simulink model "family_5_variant_2_AR_Drone_Host_Receive"  (R2014a)
settings: Solver=FixedStepDiscrete  StartTime=0.0  StopTime=inf  FixedStep=1/400  RelTol=1e-3
libraries: vrlib x3, dspnetwork x3, aerolibtransform2 x3, aerolibutil x1
settings Model: Creator=nraman  LastModifiedBy=Raphaël

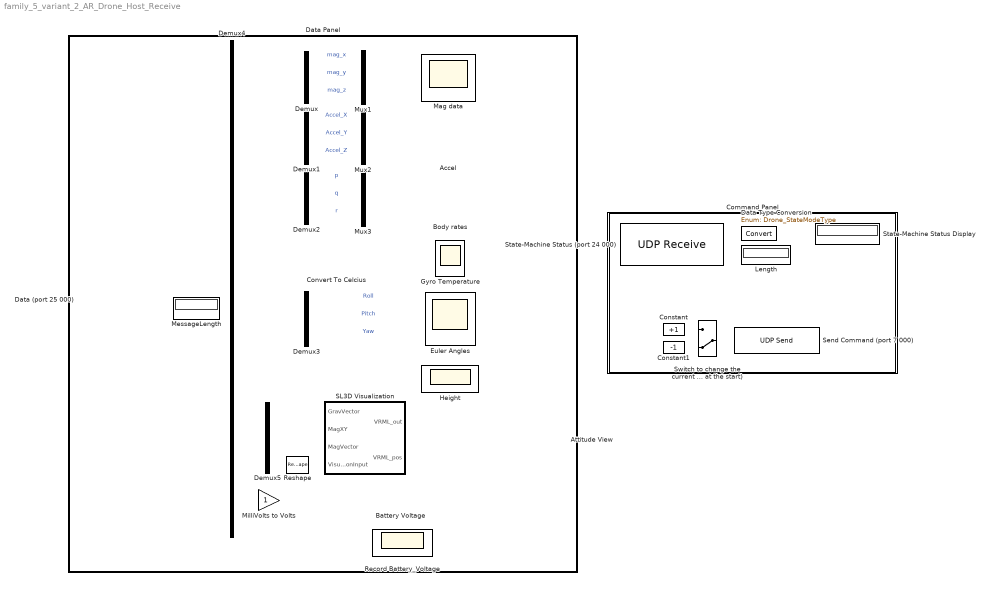
== system family_5_variant_2_AR_Drone_Host_Receive ==
  Accel : Scope
      settings: ShowLegends=on  TimeRange=100  YMin=2025  YMax=2575  SaveName=Accel
  Attitude View : vrlib/VR Sink  InstantiateOnLoad=on  SampleTime=-1  ViewEnable=on  RemoteChange=off  RemoteView=off  FieldsWritten=Drone.rotation.4.1.1.double#Drone.translation.3.1.1.double  WorldFileName=myDrone3.wrl  AutoView=off  VideoDimensions=[]  AllowVariableSize=off
  Battery Voltage : Display
  Body rates : Scope
      settings: ShowLegends=on  TimeRange=90  YMin=-45  YMax=35  SaveName=Gyro
  Command Panel : Subsystem
  Constant : Constant  Value=+1
  Constant1 : Constant  Value=-1
  Convert To Celcius : Subsystem
  Data (port 25 000) : dspnetwork/UDP Receive  localURL='0.0.0.0'  localPort=25000  remoteURL='192.168.1.1'  remotePort=-1  recvBufferSize=8192  dims=34  signalDatatype=double  isVarSize=off  showBlockingTime=off  blockingTime=0  sampletime=2/400
  Data Panel : Subsystem
  Data Type Conversion : DataTypeConversion  OutDataTypeStr=Enum: Drone_StateModeType
  Demux{,1..3} (4 alike) : Demux  Outputs=3
  Demux4 : Demux  Outputs=[3 3 3 1 3 2 18 1]
  Demux5 : Demux  Outputs=[3 3 3 9]
  Euler Angles : Scope  NumInputPorts=3
      settings: TimeRange=160  YMin=-1.04~-0.28~4.15  YMax=-0.87~-0.18~4.95  SaveName=EulerAngles
  Gyro Temperature : Scope
      settings: ShowLegends=on  TimeRange=100  YMin=47.5  YMax=82.5  SaveName=TempMeasure
  Height : Scope
      settings: YMin=-30  YMax=150  SaveName=RecordedHeight
  Length : Display
  Mag data : Scope
      settings: ShowLegends=on  TimeRange=100  YMin=-240  YMax=-30  SaveName=MagData
  MessageLength : Display
  MilliVolts to Volts : Gain
  Mux1 : Mux  Inputs=3
  Mux2 : Mux  Inputs=3
  Mux3 : Mux  Inputs=3
  Record Battery_Voltage : Scope
      settings: YMin=12.395  YMax=12.455
  Reshape : Reshape  OutputDimensionality=Customize  OutputDimensions=[3,3]
  SL3D Visualization : Subsystem
  Send Command (port 7 000) : dspnetwork/UDP Send  remoteURL='192.168.1.1'  remotePort=6000  localURL='0.0.0.0'  localPortSource=Automatically determine  localPort=-1  sampletime=-1  blockPlatform=LINUX  separateLengthPort=0
  State-Machine Status (port 24 000) : dspnetwork/UDP Receive  localURL='0.0.0.0'  localPort=24000  remoteURL='192.168.1.1'  remotePort=-1  recvBufferSize=100  dims=1  signalDatatype=int8  isVarSize=off  showBlockingTime=on  blockingTime=0.05  sampletime=1/400  blockPlatform=LINUX
  State-Machine Status Display : Display
  Switch to change the current Drone State (it has to be down at the start) : ManualSwitch  CurrentSetting=0
  wires:
  Demux4/1 -> Demux/1
  Demux/1 -> Mux1/1  "mag_x"
  Demux/2 -> Mux1/2  "mag_y"
  Demux/3 -> Mux1/3  "mag_z"
  Mux1/1 -> Mag data/1
  Demux2/1 -> Mux3/1  "p"
  Demux2/2 -> Mux3/2  "q"
  Mux3/1 -> Body rates/1
  Demux2/3 -> Mux3/3  "r"
  Demux4/3 -> Demux2/1
  Demux1/1 -> Mux2/1  "Accel_X"
  Demux1/2 -> Mux2/2  "Accel_Y"
  Mux2/1 -> Accel/1
  Demux1/3 -> Mux2/3  "Accel_Z"
  Demux4/2 -> Demux1/1
  Demux3/1 -> Euler Angles/1  "Roll"
  Demux3/2 -> Euler Angles/2  "Pitch"
  Demux4/5 -> Demux3/1
  Data (port 25 000)/1 -> Demux4/1
  MilliVolts to Volts/1 -> Battery Voltage/1, Record Battery_Voltage/1
  Demux3/3 -> Euler Angles/3  "Yaw"
  Data (port 25 000)/2 -> MessageLength/1
  State-Machine Status (port 24 000)/1 -> Data Type Conversion/1
  Data Type Conversion/1 -> State-Machine Status Display/1
  State-Machine Status (port 24 000)/2 -> Length/1
  Demux4/8 -> MilliVolts to Volts/1
  Demux4/4 -> Convert To Celcius/1(In1)
  Convert To Celcius/1(Out1) -> Gyro Temperature/1
  SL3D Visualization/1(VRML_out) -> Attitude View/1
  SL3D Visualization/2(VRML_pos) -> Attitude View/2
  Reshape/1 -> SL3D Visualization/4(VisualizationInput)
  Demux4/6 -> Height/1
  Switch to change the current Drone State (it has to be down at the start)/1 -> Send Command (port 7 000)/1
  Constant/1 -> Switch to change the current Drone State (it has to be down at the start)/1
  Constant1/1 -> Switch to change the current Drone State (it has to be down at the start)/2
  Demux5/1 -> SL3D Visualization/1(GravVector)
  Demux5/2 -> SL3D Visualization/2(MagXY)
  Demux5/3 -> SL3D Visualization/3(MagVector)
  Demux5/4 -> Reshape/1
  Demux4/7 -> Demux5/1

== system family_5_variant_2_AR_Drone_Host_Receive/Command Panel ==

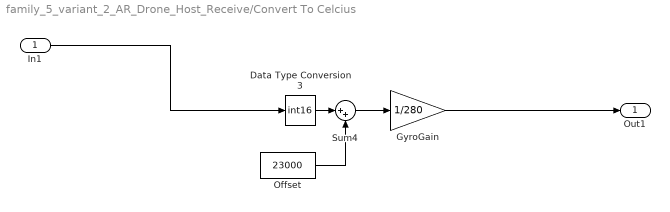
== system family_5_variant_2_AR_Drone_Host_Receive/Convert To Celcius ==
  In1 : Inport
  Data Type Conversion3 : DataTypeConversion  OutDataTypeStr=int16
  GyroGain : Gain  Gain=1/280  OutDataTypeStr=double
  Offset : Constant  Value=23000  OutDataTypeStr=int16
  Sum4 : Sum  Inputs=|++
  Out1 : Outport
  wires:
  Offset/1 -> Sum4/2
  Sum4/1 -> GyroGain/1
  GyroGain/1 -> Out1/1
  In1/1 -> Data Type Conversion3/1
  Data Type Conversion3/1 -> Sum4/1

== system family_5_variant_2_AR_Drone_Host_Receive/Data Panel ==

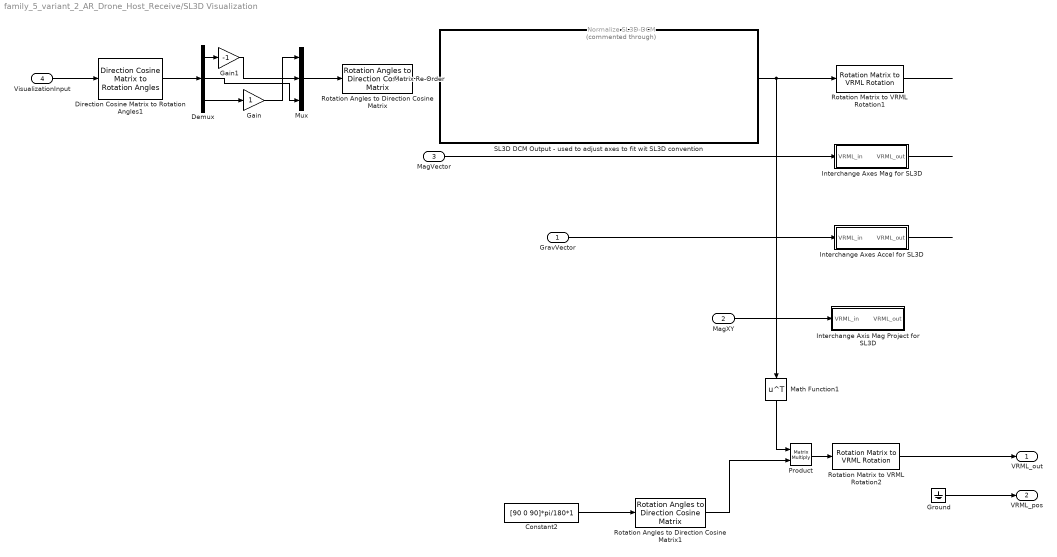
== system family_5_variant_2_AR_Drone_Host_Receive/SL3D Visualization ==
  GravVector : Inport
  MagXY : Inport  Port=2
  MagVector : Inport  Port=3
  VisualizationInput : Inport  Port=4
  Constant2 : Constant  Value=[90 0 90]*pi/180*1
  Demux : Demux  Outputs=3
  Direction Cosine Matrix to Rotation Angles1 : aerolibtransform2/Direction Cosine Matrix to Rotation Angles  rotationOrder=XYZ  lim=ZeroR3
      settings: AttributesFormatString=Rotation Order: %<rotationOrder>
  Gain : Gain  OutDataTypeStr=Inherit: Same as input
  Gain1 : Gain  Gain=-1  OutDataTypeStr=Inherit: Same as input
  Ground : Ground
  "Interchange Axes Accel for SL3D " : Subsystem
  "Interchange Axes Mag for SL3D " : Subsystem
  Interchange Axis Mag Project for SL3D : Subsystem
  Math Function1 : Math  Operator=transpose  SaturateOnIntegerOverflow=on
  Matrix Re-Order : MATLAB Function  TreatAsAtomicUnit=on
  Mux : Mux  Inputs=3
  Normalize SL3D-DCM : Subsystem  Commented=through  TreatAsAtomicUnit=on
  Product : Product  Multiplication=Matrix(*)
  Rotation Angles to Direction Cosine Matrix : aerolibtransform2/Rotation Angles to Direction Cosine Matrix  rotationOrder=XYZ
  Rotation Angles to Direction Cosine Matrix1 : aerolibtransform2/Rotation Angles to Direction Cosine Matrix  rotationOrder=XYZ
  Rotation Matrix to VRML Rotation1 : vrlib/Utilities/Rotation Matrix to VRML Rotation  maxzero=1e-12
  Rotation Matrix to VRML Rotation2 : vrlib/Utilities/Rotation Matrix to VRML Rotation  maxzero=1e-12
  SL3D DCM Output - used to adjust axes to fit wit SL3D convention : Subsystem
  VRML_out : Outport
  VRML_pos : Outport  Port=2
  wires:
  Rotation Matrix to VRML Rotation1/1 -> ?
  "Interchange Axes Accel for SL3D "/1(VRML_out) -> ?
  VisualizationInput/1 -> Direction Cosine Matrix to Rotation Angles1/1
  GravVector/1 -> "Interchange Axes Accel for SL3D "/1(VRML_in)
  Matrix Re-Order/1(M_out) -> Normalize SL3D-DCM/1(DCM)
  Direction Cosine Matrix to Rotation Angles1/1 -> Demux/1
  Demux/3 -> Gain/1
  Mux/1 -> Rotation Angles to Direction Cosine Matrix/1
  "Interchange Axes Mag for SL3D "/1(VRML_out) -> ?
  MagVector/1 -> "Interchange Axes Mag for SL3D "/1(VRML_in)
  Rotation Angles to Direction Cosine Matrix/1 -> Matrix Re-Order/1(M_in)
  MagXY/1 -> Interchange Axis Mag Project for SL3D/1(VRML_in)
  Rotation Matrix to VRML Rotation2/1 -> VRML_out/1
  Constant2/1 -> Rotation Angles to Direction Cosine Matrix1/1
  Rotation Angles to Direction Cosine Matrix1/1 -> Product/2
  Product/1 -> Rotation Matrix to VRML Rotation2/1
  Normalize SL3D-DCM/1(DCM_normalized) -> Math Function1/1, Rotation Matrix to VRML Rotation1/1
  Math Function1/1 -> Product/1
  Gain/1 -> Mux/1
  Demux/1 -> Gain1/1
  Demux/2 -> Mux/3
  Gain1/1 -> Mux/2
  Ground/1 -> VRML_pos/1

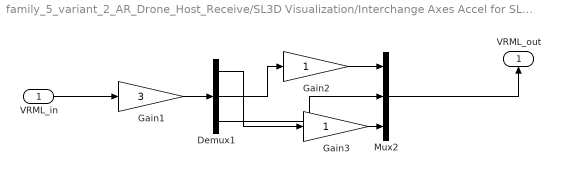
== system family_5_variant_2_AR_Drone_Host_Receive/SL3D Visualization/Interchange Axes Accel for SL3D  ==
  VRML_in : Inport
  Demux1 : Demux  Outputs=3
  Gain1 : Gain  Gain=3
  Gain2 : Gain
  Gain3 : Gain
  Mux2 : Mux  Inputs=3
  VRML_out : Outport
  wires:
  Gain1/1 -> Demux1/1
  Demux1/1 -> Gain3/1
  Demux1/3 -> Mux2/2
  Gain2/1 -> Mux2/1
  Gain3/1 -> Mux2/3
  Mux2/1 -> VRML_out/1
  Demux1/2 -> Gain2/1
  VRML_in/1 -> Gain1/1

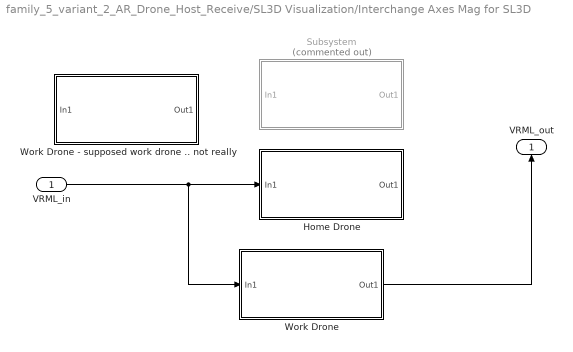
== system family_5_variant_2_AR_Drone_Host_Receive/SL3D Visualization/Interchange Axes Mag for SL3D  ==
  VRML_in : Inport
  Home Drone : Subsystem
  Subsystem : Subsystem  Commented=on
  Work Drone : Subsystem
  Work Drone - supposed work drone .. not really : Subsystem
  VRML_out : Outport
  wires:
  VRML_in/1 -> Work Drone/1(In1), Home Drone/1(In1)
  Work Drone/1(Out1) -> VRML_out/1

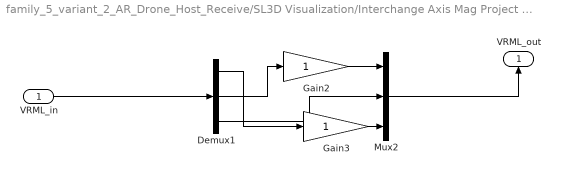
== system family_5_variant_2_AR_Drone_Host_Receive/SL3D Visualization/Interchange Axis Mag Project for SL3D ==
  VRML_in : Inport
  Demux1 : Demux  Outputs=3
  Gain2 : Gain
  Gain3 : Gain
  Mux2 : Mux  Inputs=3
  VRML_out : Outport
  wires:
  VRML_in/1 -> Demux1/1
  Demux1/1 -> Gain3/1
  Demux1/3 -> Mux2/2
  Gain2/1 -> Mux2/1
  Gain3/1 -> Mux2/3
  Mux2/1 -> VRML_out/1
  Demux1/2 -> Gain2/1

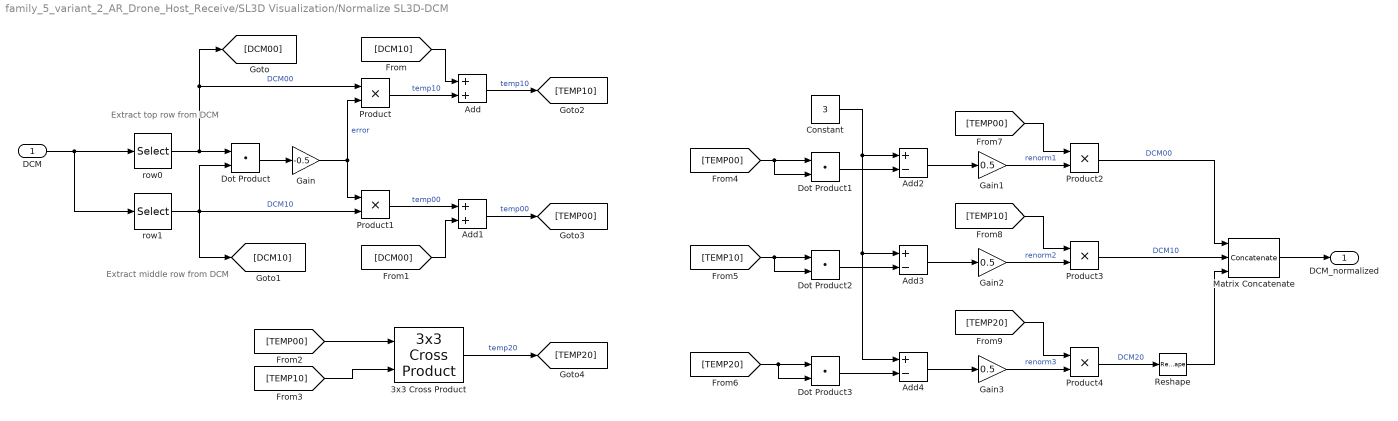
== system family_5_variant_2_AR_Drone_Host_Receive/SL3D Visualization/Normalize SL3D-DCM ==
  note: Extract middle row from DCM
  note: Extract top row from DCM
  DCM : Inport  OutDataTypeStr=double  PortDimensions=[3,3]
  3x3 Cross Product : aerolibutil/3x3 Cross Product
  Add : Sum
  Add1 : Sum
  Add2 : Sum  Inputs=+-
  Add3 : Sum  Inputs=+-
  Add4 : Sum  Inputs=+-
  Constant : Constant  Value=3  OutDataTypeStr=double  SampleTime=-1
  Dot Product{,1..3} (4 alike) : DotProduct  InputSameDT=on  OutDataTypeStr=Inherit: Inherit via internal rule
  Gain : Gain  Gain=-0.5
  Gain1 : Gain  Gain=0.5  OutDataTypeStr=single
  Gain2 : Gain  Gain=0.5  OutDataTypeStr=single
  Gain3 : Gain  Gain=0.5  OutDataTypeStr=single
  Matrix Concatenate : Concatenate  NumInputs=3  Mode=Multidimensional array
  Product{,1..4} (5 alike) : Product  RndMeth=Zero
  Reshape : Reshape  OutputDimensionality=Row vector (2-D)
  row0 : Selector  NumberOfDimensions=2  IndexMode=Zero-based  InputPortWidth=3  IndexOptions=Index vector (dialog),Index vector (dialog)  Indices=0,[0:2]  OutputSizes=1,1
  row1 : Selector  NumberOfDimensions=2  IndexMode=Zero-based  InputPortWidth=3  IndexOptions=Index vector (dialog),Index vector (dialog)  Indices=1,[0:2]  OutputSizes=1,1
  DCM_normalized : Outport  OutDataTypeStr=double
  wires:
  Reshape/1 -> Matrix Concatenate/3
  Matrix Concatenate/1 -> DCM_normalized/1
  Product4/1 -> Reshape/1  "DCM20"
  Product3/1 -> Matrix Concatenate/2  "DCM10"
  Product2/1 -> Matrix Concatenate/1  "DCM00"
  [TEMP20] -> Product4/1
  [TEMP10] -> Product3/1
  [TEMP00] -> Product2/1
  Dot Product3/1 -> Add4/2
  Gain3/1 -> Product4/2  "renorm3"
  Add4/1 -> Gain3/1
  Dot Product2/1 -> Add3/2
  Gain2/1 -> Product3/2  "renorm2"
  Add3/1 -> Gain2/1
  Gain1/1 -> Product2/2  "renorm1"
  Add2/1 -> Gain1/1
  Constant/1 -> Add3/1, Add4/1, Add2/1
  Dot Product1/1 -> Add2/2
  [TEMP20] -> Dot Product3/2, Dot Product3/1
  [TEMP10] -> Dot Product2/2, Dot Product2/1
  [TEMP00] -> Dot Product1/2, Dot Product1/1
  [TEMP10] -> 3x3 Cross Product/2
  [TEMP00] -> 3x3 Cross Product/1
  3x3 Cross Product/1 -> [TEMP20]  "temp20"
  Add1/1 -> [TEMP00]  "temp00"
  Add/1 -> [TEMP10]  "temp10"
  [DCM00] -> Add1/2
  [DCM10] -> Add/1
  Product1/1 -> Add1/1  "temp00"
  Product/1 -> Add/2  "temp10"
  Gain/1 -> Product1/1, Product/2  "error"
  Dot Product/1 -> Gain/1
  row1/1 -> [DCM10], Product1/2, Dot Product/2  "DCM10"
  row0/1 -> [DCM00], Product/1, Dot Product/1  "DCM00"
  DCM/1 -> row1/1, row0/1

== system family_5_variant_2_AR_Drone_Host_Receive/SL3D Visualization/SL3D DCM Output - used to adjust axes to fit wit SL3D convention ==

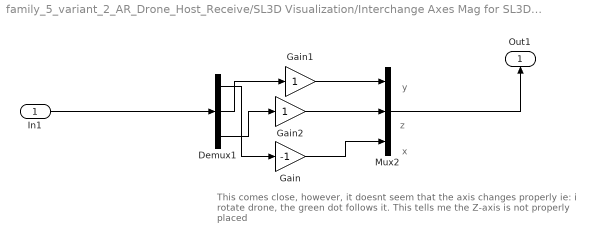
== system family_5_variant_2_AR_Drone_Host_Receive/SL3D Visualization/Interchange Axes Mag for SL3D /Home Drone ==
  note: This comes close, however, it doesnt seem that the axis changes properly
      | ie: i rotate drone, the green dot follows it. This  tells me the Z-axis is not
      |  properly placed
  note: y
  note: x
  note: z
  In1 : Inport
  Demux1 : Demux  Outputs=3
  Gain : Gain  Gain=-1
  Gain1 : Gain
  Gain2 : Gain
  Mux2 : Mux  Inputs=3
  Out1 : Outport
  wires:
  Mux2/1 -> Out1/1
  In1/1 -> Demux1/1
  Demux1/3 -> Gain2/1
  Gain2/1 -> Mux2/2
  Demux1/1 -> Gain/1
  Gain/1 -> Mux2/3
  Demux1/2 -> Gain1/1
  Gain1/1 -> Mux2/1

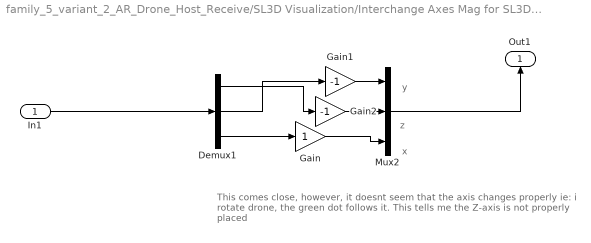
== system family_5_variant_2_AR_Drone_Host_Receive/SL3D Visualization/Interchange Axes Mag for SL3D /Subsystem ==
  note: This comes close, however, it doesnt seem that the axis changes properly
      | ie: i rotate drone, the green dot follows it. This  tells me the Z-axis is not
      |  properly placed
  note: y
  note: x
  note: z
  In1 : Inport
  Demux1 : Demux  Outputs=3
  Gain : Gain
  Gain1 : Gain  Gain=-1
  Gain2 : Gain  Gain=-1
  Mux2 : Mux  Inputs=3
  Out1 : Outport
  wires:
  Demux1/1 -> Gain2/1
  Gain2/1 -> Mux2/2
  Gain/1 -> Mux2/3
  Gain1/1 -> Mux2/1
  Mux2/1 -> Out1/1
  Demux1/2 -> Gain1/1
  Demux1/3 -> Gain/1
  In1/1 -> Demux1/1

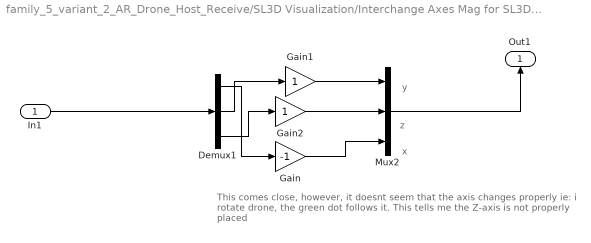
== system family_5_variant_2_AR_Drone_Host_Receive/SL3D Visualization/Interchange Axes Mag for SL3D /Work Drone ==
  note: This comes close, however, it doesnt seem that the axis changes properly
      | ie: i rotate drone, the green dot follows it. This  tells me the Z-axis is not
      |  properly placed
  note: y
  note: x
  note: z
  In1 : Inport
  Demux1 : Demux  Outputs=3
  Gain : Gain  Gain=-1
  Gain1 : Gain
  Gain2 : Gain
  Mux2 : Mux  Inputs=3
  Out1 : Outport
  wires:
  Mux2/1 -> Out1/1
  In1/1 -> Demux1/1
  Demux1/3 -> Gain2/1
  Gain2/1 -> Mux2/2
  Demux1/1 -> Gain/1
  Gain/1 -> Mux2/3
  Demux1/2 -> Gain1/1
  Gain1/1 -> Mux2/1

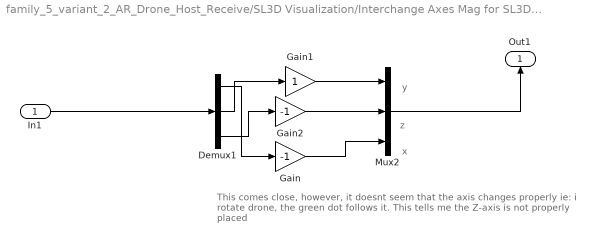
== system family_5_variant_2_AR_Drone_Host_Receive/SL3D Visualization/Interchange Axes Mag for SL3D /Work Drone - supposed work drone .. not really ==
  note: This comes close, however, it doesnt seem that the axis changes properly
      | ie: i rotate drone, the green dot follows it. This  tells me the Z-axis is not
      |  properly placed
  note: y
  note: x
  note: z
  In1 : Inport
  Demux1 : Demux  Outputs=3
  Gain : Gain  Gain=-1
  Gain1 : Gain
  Gain2 : Gain  Gain=-1
  Mux2 : Mux  Inputs=3
  Out1 : Outport
  wires:
  Mux2/1 -> Out1/1
  In1/1 -> Demux1/1
  Demux1/3 -> Gain2/1
  Gain2/1 -> Mux2/2
  Demux1/1 -> Gain/1
  Gain/1 -> Mux2/3
  Demux1/2 -> Gain1/1
  Gain1/1 -> Mux2/1

== matlab function family_5_variant_2_AR_Drone_Host_Receive/SL3D Visualization/Matrix Re-Order ==
  data: M_in input; M_out output
function M_out = MatrixFormat(M_in)
%#codegen

% SL3D coordinate system is different. This EML block is responsible for
% re-ordering the matrix in a format that SL3D can understand

M_out = M_in ; %set size

%re-order diagonal
M_out(1,1) = M_in(2,2);
M_out(2,2) = M_in(3,3);
M_out(3,3) = M_in(1,1);

%re-order bottom half
M_out(2,1) = M_in(3,2) ;
M_out(3,1) = M_in(1,2) ;
M_out(3,2) = M_in(1,3);

%re-order upper half
M_out(1,2) = M_in(2,3);
M_out(1,3) = M_in(2,1) ;
M_out(2,3) = M_in(3,1);
